simulink model "function3"  (R2020b)
settings: Solver=VariableStepAuto  StartTime=0.0  StopTime=10.0  RelTol=1e-3
settings Model: Creator=Aurelie  LastModifiedBy=Aurelie

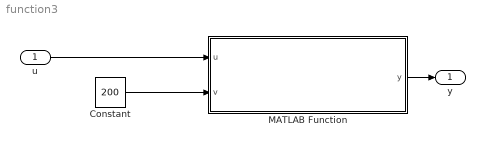
== system function3 ==
  u : Inport
  Constant : Constant  Value=200
  MATLAB Function : MATLAB Function  TreatAsAtomicUnit=on
  y : Outport
  wires:
  MATLAB Function/1(y) -> y/1
  u/1 -> MATLAB Function/1(u)
  Constant/1 -> MATLAB Function/2(v)

== matlab function function3/MATLAB Function ==
  data: u input; y output; v input
function y = calladition(u,v)
y = adition(u,v);
end
